simulink model "transmit_test"  (R2024b)
settings: Solver=FixedStepAuto  StartTime=0.0  StopTime=0  FixedStep=1  RelTol=1e-3
values from neighbouring files (symbols this model uses):
  RandomizeSequence = hexToArray(RandomizeSequence,0)    [Full_transmit.m]
  SBStream = hexToArray(SBStream,1)    [Full_transmit.m]
libraries: simulink x5, commcnvcod2 x1, commblkintrlv2 x1
settings Model: Creator=fredr  LastModifiedBy=fredr

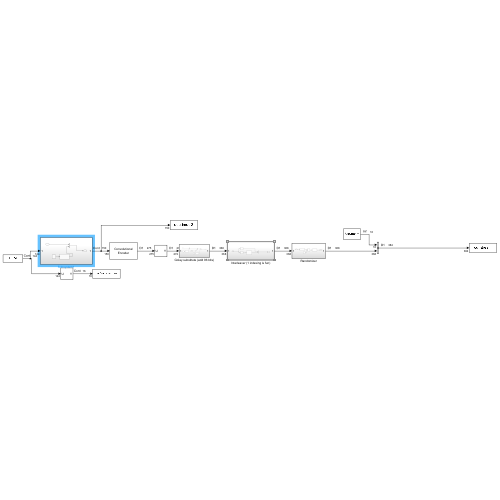
[thumbnail: Simulink's stored preview of the top-level diagram]
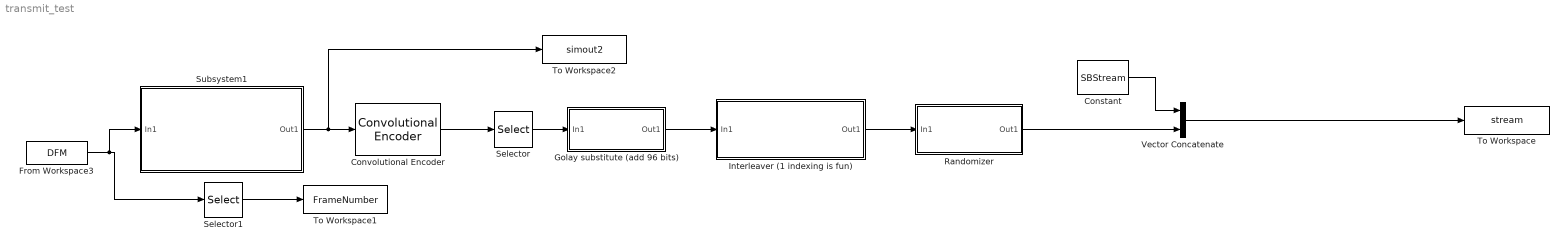
== system transmit_test ==
  Constant : Constant  Value=SBStream
  Convolutional Encoder : commcnvcod2/Convolutional Encoder  trellis=poly2trellis(5, [23 35])  opMode=Continuous  DelayedResetAction=on  hasIniStPort=off  hasFinStPort=off  usePuncVector=on  punctureVector=P2  reset=Unused parameter value
      settings: LibrarySourceBlock=|
      | commhdlcnvcod/Convolutional
      | Encoder
  From Workspace3 : FromWorkspace  VariableName=DFM  Interpolate=off  OutputAfterFinalValue=Setting to zero
  Golay substitute (add 96 bits) : Subsystem
  Interleaver (1 indexing is fun) : Subsystem
  Randomizer : Subsystem
  Selector : Selector  IndexOptions=Index vector (dialog)  Indices=[1:272]  OutputSizes=1
  Selector1 : Selector  IndexOptions=Index vector (dialog)  Indices=[129:144]  OutputSizes=1
  Subsystem1 : Subsystem
  To Workspace : ToWorkspace  VariableName=stream  SampleTime=-1
      settings: Save2DSignal=2-D array (concatenate along first dimension)
  To Workspace1 : ToWorkspace  VariableName=FrameNumber  SampleTime=-1
      settings: Save2DSignal=2-D array (concatenate along first dimension)
  To Workspace2 : ToWorkspace  VariableName=simout2  SampleTime=-1
      settings: Save2DSignal=2-D array (concatenate along first dimension)
  Vector Concatenate : Concatenate
  wires:
  Interleaver (1 indexing is fun)/1(Out1) -> Randomizer/1(In1)
  Selector/1 -> Golay substitute (add 96 bits)/1(In1)
  Convolutional Encoder/1 -> Selector/1
  Golay substitute (add 96 bits)/1(Out1) -> Interleaver (1 indexing is fun)/1(In1)
  Vector Concatenate/1 -> To Workspace/1
  Selector1/1 -> To Workspace1/1
  From Workspace3/1 -> Subsystem1/1(In1), Selector1/1
  Subsystem1/1(Out1) -> Convolutional Encoder/1, To Workspace2/1
  Constant/1 -> Vector Concatenate/1
  Randomizer/1(Out1) -> Vector Concatenate/2

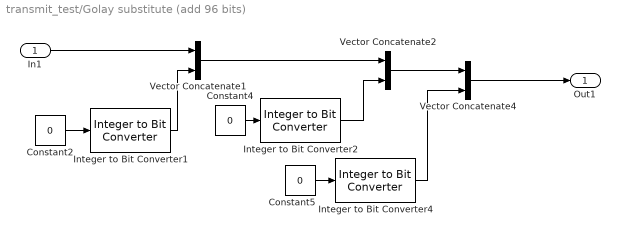
== system transmit_test/Golay substitute (add 96 bits) ==
  In1 : Inport
  Constant2 : Constant  Value=0
  Constant4 : Constant  Value=0
  Constant5 : Constant  Value=0
  Integer to Bit Converter1 : simulink/Logic and Bit Operations/Integer to Bit Converter  nbits=32  signedInputValues=Unsigned  bitOrder=MSB first  outDtype=Inherit via internal rule
  Integer to Bit Converter2 : simulink/Logic and Bit Operations/Integer to Bit Converter  nbits=32  signedInputValues=Unsigned  bitOrder=MSB first  outDtype=Inherit via internal rule
  Integer to Bit Converter4 : simulink/Logic and Bit Operations/Integer to Bit Converter  nbits=32  signedInputValues=Unsigned  bitOrder=MSB first  outDtype=Inherit via internal rule
  Vector Concatenate1 : Concatenate
  Vector Concatenate2 : Concatenate
  Vector Concatenate4 : Concatenate
  Out1 : Outport
  wires:
  Integer to Bit Converter4/1 -> Vector Concatenate4/2
  Constant5/1 -> Integer to Bit Converter4/1
  Integer to Bit Converter2/1 -> Vector Concatenate2/2
  Integer to Bit Converter1/1 -> Vector Concatenate1/2
  Constant4/1 -> Integer to Bit Converter2/1
  Constant2/1 -> Integer to Bit Converter1/1
  In1/1 -> Vector Concatenate1/1
  Vector Concatenate1/1 -> Vector Concatenate2/1
  Vector Concatenate2/1 -> Vector Concatenate4/1
  Vector Concatenate4/1 -> Out1/1

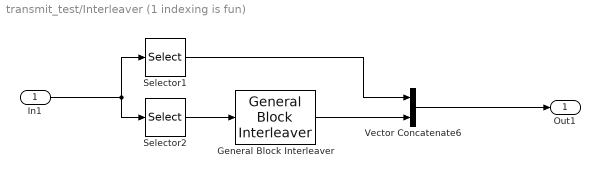
== system transmit_test/Interleaver (1 indexing is fun) ==
  In1 : Inport
  General Block Interleaver : commblkintrlv2/General Block Interleaver  StatePerturbationForJacobian=1.0e-05  permutationVectorSource=Dialog  elements=InterleavingVector
  Selector1 : Selector  IndexOptions=Index vector (dialog)  Indices=[1]  OutputSizes=1
  Selector2 : Selector  IndexOptions=Index vector (dialog)  Indices=[2:368]  OutputSizes=1
  Vector Concatenate6 : Concatenate
  Out1 : Outport
  wires:
  General Block Interleaver/1 -> Vector Concatenate6/2
  Selector1/1 -> Vector Concatenate6/1
  In1/1 -> Selector2/1, Selector1/1
  Selector2/1 -> General Block Interleaver/1
  Vector Concatenate6/1 -> Out1/1

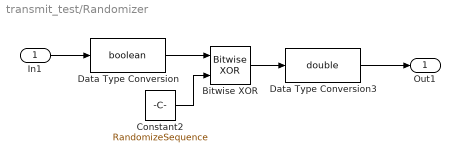
== system transmit_test/Randomizer ==
  In1 : Inport
  Bitwise XOR : simulink/Logic and Bit Operations/Bitwise Operator  logicop=XOR  UseBitMask=off  NumInputPorts=2  BitMask=bin2dec('11011001')  BitMaskRealWorld=Stored Integer
  Constant2 : Constant  Value=RandomizeSequence
  Data Type Conversion : DataTypeConversion  OutDataTypeStr=boolean  SaturateOnIntegerOverflow=off  RndMeth=Floor
  Data Type Conversion3 : DataTypeConversion  OutDataTypeStr=double  SaturateOnIntegerOverflow=off  RndMeth=Floor
  Out1 : Outport
  wires:
  Data Type Conversion/1 -> Bitwise XOR/1
  Data Type Conversion3/1 -> Out1/1
  In1/1 -> Data Type Conversion/1
  Constant2/1 -> Bitwise XOR/2
  Bitwise XOR/1 -> Data Type Conversion3/1

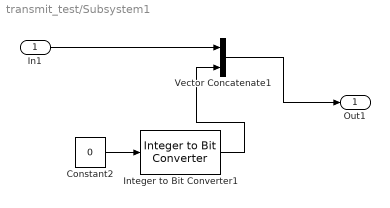
== system transmit_test/Subsystem1 ==
  In1 : Inport
  Constant2 : Constant  Value=0
  Integer to Bit Converter1 : simulink/Logic and Bit Operations/Integer to Bit Converter  nbits=6  signedInputValues=Unsigned  bitOrder=MSB first  outDtype=Inherit via internal rule
  Vector Concatenate1 : Concatenate
  Out1 : Outport
  wires:
  Vector Concatenate1/1 -> Out1/1
  Constant2/1 -> Integer to Bit Converter1/1
  Integer to Bit Converter1/1 -> Vector Concatenate1/2
  In1/1 -> Vector Concatenate1/1
